simulink library "LCDScope"  (R2015a)
settings: Solver=ode45  StartTime=0.0  StopTime=10.0  RelTol=1e-3
libraries: mbed_lib x1
settings Model: CovSFcnEnable=off  Creator=Schlueter  LastModifiedBy=oh
settings DebuggingCC: SolverPrmCheckMsg=warning

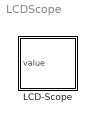
== system LCDScope ==
  LCD-Scope : Subsystem  mask(LCD-Scope){MinValue=0, MaxValue=120, StepSize=1, TimeRange=500, scaleValue=1e0}
      mask prompts: MinValue "Min Value"; MaxValue "Max Value"; StepSize "Step Size"; TimeRange "Samples per Window"; scaleValue "Scale Value"
      mask help:
      | Dieser Block kann genutzt werden um Signale mit dem LCD Mi0283QT darzustellen.
      | Für die Kommunikation wird SPI verwendet. Die verwendeten PINs lassen sich innerhalb des Blocks einstellen und ändern.
      mask init:
      | StepSize = 1;
      mask Display: disp('Scope')

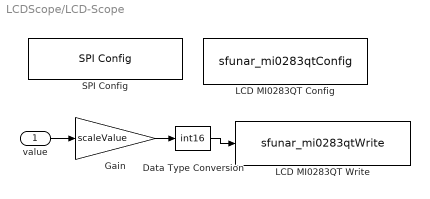
== system LCDScope/LCD-Scope ==
  value : Inport
  Data Type Conversion : DataTypeConversion  OutDataTypeStr=int16
  Gain : Gain  Gain=scaleValue
  LCD MI0283QT Config : S-Function  Priority=0  FunctionName=sfunar_mi0283qtConfig  Parameters=uint8(0), uint8(MOSI_PORT), uint8(MOSI_PIN), uint8(MISO_PORT), uint8(MISO_PIN), SPI_FREQ, uint8(SCK_PORT), uint8(SCK_PIN), uint8(CS_PORT), uint8(CS_PIN), uint8(RST_PORT), uint8(RST_PIN)  mask(LCD MI0283QT Configuration){SPI_FREQ=8000000, MOSI_PORT=B, MOSI_PIN=5, MISO_PORT=B, MISO_PIN=4, SCK_PORT=B, SCK_PIN=3, CS_PORT=B, CS_PIN=11, RST_PORT=B, RST_PIN=10}
      mask prompts: SPI_FREQ "Bus frequency: [Hz]"; MOSI_PORT "MOSI: Port"; MOSI_PIN "Pin"; MISO_PORT "MISO: Port"; MISO_PIN "Pin"; SCK_PORT "SCK: Port"; SCK_PIN "Pin"; CS_PORT "CS: Port"; CS_PIN "Pin"; RST_PORT "RST: Port"; RST_PIN "Pin"
      mask help: This blocks sets up the SPI connection on the mbed board to LCD Mi0283QT.
      mask TypeOptions MOSI_PORT: A | B | C | D | E | F
      mask TypeOptions MOSI_PIN: 0 | 1 | 2 | 3 | 4 | 5 | 6 | 7 | 8 | 9 | 10 | 11 | 12 | 13 | 14 | 15
      mask TypeOptions MISO_PORT: A | B | C | D | E | F
      mask TypeOptions MISO_PIN: 0 | 1 | 2 | 3 | 4 | 5 | 6 | 7 | 8 | 9 | 10 | 11 | 12 | 13 | 14 | 15
      mask TypeOptions SCK_PORT: A | B | C | D | E | F
      mask TypeOptions SCK_PIN: 0 | 1 | 2 | 3 | 4 | 5 | 6 | 7 | 8 | 9 | 10 | 11 | 12 | 13 | 14 | 15
      mask TypeOptions CS_PORT: A | B | C | D | E | F
      mask TypeOptions CS_PIN: 0 | 1 | 2 | 3 | 4 | 5 | 6 | 7 | 8 | 9 | 10 | 11 | 12 | 13 | 14 | 15
      mask TypeOptions RST_PORT: A | B | C | D | E | F
      mask TypeOptions RST_PIN: 0 | 1 | 2 | 3 | 4 | 5 | 6 | 7 | 8 | 9 | 10 | 11 | 12 | 13 | 14 | 15
      mask Display:
      | disp(['\nMOSI: ' MOSI_PORT+64 '.' num2str(MOSI_PIN-1) ', MISO: ' MISO_PORT+64, '.' num2str(MISO_PIN-1)  ', SCK: ' SCK_PORT+64, '.' num2str(SCK_PIN-1) ' \n\n\n']);
      | disp(['\nCS: ' CS_PORT+64 '.' num2str(CS_PIN-1) ', RST: ' RST_PORT+64, '.' num2str(RST_PIN-1) ' \n']);
      | disp(['\n\nFrequency: ' num2str(SPI_FREQ) ' HZ']);
  LCD MI0283QT Write : S-Function  FunctionName=sfunar_mi0283qtWrite  Parameters=int16(MinValue), int16(MaxValue), uint16(StepSize), uint16(TimeRange)  mask(Draw Value on LCD-Scope){SPIPort=1, CSPort=B, CSPin=11, RSTPort=B, RSTPin=10, MinValue=MinValue*scaleValue, MaxValue=MaxValue*scaleValue, StepSize=StepSize, TimeRange=TimeRange}
      mask prompts: SPIPort "SPI Port"; CSPort "CS: Port"; CSPin "Pin"; RSTPort "RST: Port"; RSTPin "Pin"; MinValue "Min Value"; MaxValue "Max Value"; StepSize "Step Size"; TimeRange "Time Range"
      mask TypeOptions SPIPort: 1 | 2 | 3 | 4
      mask TypeOptions CSPort: A | B | C | D | E | F
      mask TypeOptions CSPin: 0 | 1 | 2 | 3 | 4 | 5 | 6 | 7 | 8 | 9 | 10 | 11 | 12 | 13 | 14 | 15
      mask TypeOptions RSTPort: A | B | C | D | E | F
      mask TypeOptions RSTPin: 0 | 1 | 2 | 3 | 4 | 5 | 6 | 7 | 8 | 9 | 10 | 11 | 12 | 13 | 14 | 15
      mask Display:
      | disp(['Write Scope' ' \n\n']);
      | disp(['\nSPI ' num2str(SPIPort) '\n']);
      | disp(['\n\n\nCS: ' CSPort+64 '.' num2str(CSPin-1) ', RST: ' RSTPort+64, '.' num2str(RSTPin-1) ' \n']);
  SPI Config : mbed_lib/SPI/SPI Config  Priority=0  SpiPort=1  SParameter6=8000000  SParameter2=B  SParameter3=5  SParameter4=B  SParameter5=4  SCK_PORT=B  SCK_PIN=3
  wires:
  value/1 -> Gain/1
  Data Type Conversion/1 -> LCD MI0283QT Write/1
  Gain/1 -> Data Type Conversion/1
